simulink model "Controller_Design_Simulink"  (R2025b)
settings: Solver=ode45  StartTime=0.0  StopTime=1  RelTol=1e-10
InitFcn:
  | load("simulink_data.mat")
StartFcn:
  | load("simulink_data.mat")
values from neighbouring files (symbols this model uses):
  A_2 = 1    [Controller_Design.m]    (also in DISTURBANCE TOLERANCE ANALYSYS 2.B.III.mat; Disturbance_tolerance_2.B.I.mat; simulink_data.mat)
  denC = [1 0 0 0]    [simulink_data.mat]
  denFf = [1 4442.21201218 9869604.40109 0]    [simulink_data.mat]
  denFr = 1    [simulink_data.mat]
  denH = [1 88.8576587632 286218.527632 12540956.142 19919185025.5]    [simulink_data.mat]
  denP = [1 1461.98844298 0.0730994152047]    [simulink_data.mat]
  f = 55    [Controller_Design.m]    (also in DISTURBANCE TOLERANCE ANALYSYS 2.B.III.mat = 60; Disturbance_tolerance_2.B.I.mat = 60; simulink_data.mat)
  numC = [0 -1 -4 -4]    [simulink_data.mat]
  numFf = [0 -1731.54607852 -2531500.35528 -126.57500574]    [simulink_data.mat]
  numFr = 1    [simulink_data.mat]
  numH = [1 0 282270.685871 0 19919185025.5]    [simulink_data.mat]
  numP = [0 -5699.87973381 0]    [simulink_data.mat]
libraries: simulink x1
settings Model: Creator=jacop  LastModifiedBy=jacop

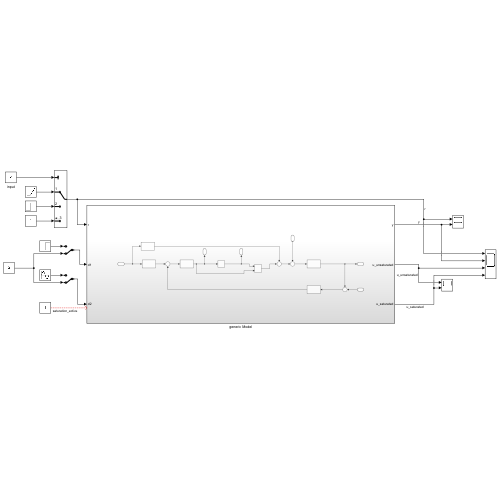
[thumbnail: Simulink's stored preview of the top-level diagram]
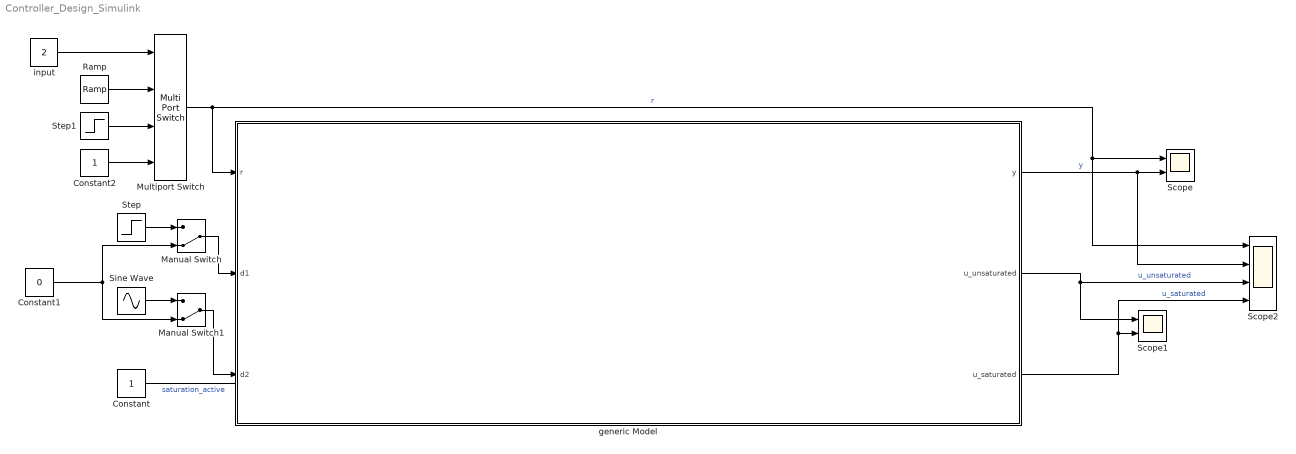
== system Controller_Design_Simulink ==
  Constant : Constant
  Constant1 : Constant  Value=0
  Constant2 : Constant
  Manual Switch : ManualSwitch  CurrentSetting=0
  Manual Switch1 : ManualSwitch  CurrentSetting=0
  Multiport Switch : MultiPortSwitch  SaturateOnIntegerOverflow=off  InputSameDT=off
  Ramp : simulink/Sources/Ramp  slope=1  start=0  InitialOutput=0
  Scope : Scope  NumInputPorts=2
      settings: ActiveDisplayYMinimum=9.9997548415478573E+9  ActiveDisplayYMaximum=1.0000142907162624E+10
  Scope1 : Scope  NumInputPorts=2
      settings: ActiveDisplayYMinimum=-18924.681476074558  ActiveDisplayYMaximum=2102.7423862305059
  Scope2 : Scope  NumInputPorts=4
      settings: ActiveDisplayYMinimum=-50312.130787861315  ActiveDisplayYMaximum=446718.69500859728  DataLoggingVariableName=ScopeData2
  Sine Wave : Sin  Amplitude=A_2  Frequency=2*pi*f  SampleTime=0
  Step : Step  SampleTime=0
  Step1 : Step  Time=0  After=1e7  SampleTime=0
  generic Model : Subsystem
  input : Constant  Value=2
  wires:
  Ramp/1 -> Multiport Switch/2
  Step/1 -> Manual Switch/1
  generic Model/1(y) -> Scope2/2, Scope/2  "y"
  Constant/1 -> ?  "saturation_active"
  generic Model/2(u_unsaturated) -> Scope1/1, Scope2/3  "u_unsaturated"
  generic Model/3(u_saturated) -> Scope2/4, Scope1/2  "u_saturated"
  Constant1/1 -> Manual Switch/2, Manual Switch1/2
  Multiport Switch/1 -> Scope2/1, Scope/1, generic Model/1(r)  "r"
  input/1 -> Multiport Switch/1
  Constant2/1 -> Multiport Switch/4
  Step1/1 -> Multiport Switch/3
  Sine Wave/1 -> Manual Switch1/1
  Manual Switch/1 -> generic Model/2(d1)
  Manual Switch1/1 -> generic Model/3(d2)

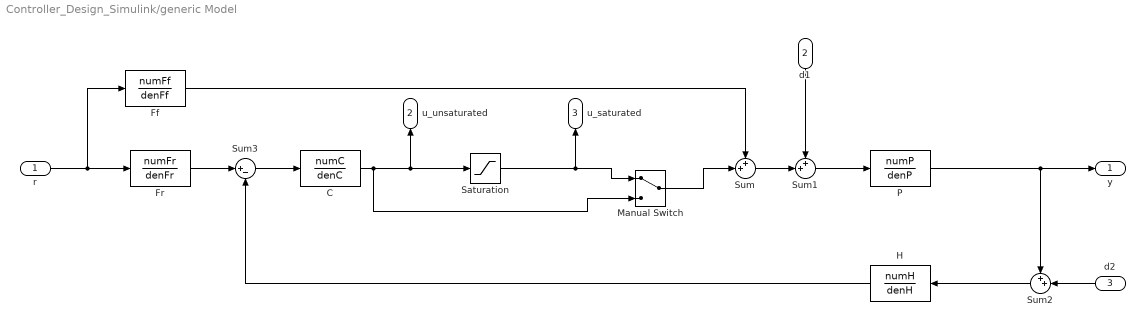
== system Controller_Design_Simulink/generic Model ==
  r : Inport
  d1 : Inport  Port=2
  d2 : Inport  Port=3
  C : TransferFcn  Numerator=numC  Denominator=denC
  Ff : TransferFcn  Numerator=numFf  Denominator=denFf
  Fr : TransferFcn  Numerator=numFr  Denominator=denFr
  H : TransferFcn  Numerator=numH  Denominator=denH
  Manual Switch : ManualSwitch
  P : TransferFcn  Numerator=numP  Denominator=denP
  Saturation : Saturate  UpperLimit=5*1000  LowerLimit=-5*1000
  Sum : Sum  Inputs=++|
  Sum1 : Sum  Inputs=++|
  Sum2 : Sum  Inputs=++|
  Sum3 : Sum  Inputs=|+-
  y : Outport
  u_unsaturated : Outport  Port=2
  u_saturated : Outport  Port=3
  wires:
  Sum2/1 -> H/1
  Ff/1 -> Sum/1
  r/1 -> Fr/1, Ff/1
  Sum1/1 -> P/1
  Sum/1 -> Sum1/2
  Sum3/1 -> C/1
  P/1 -> y/1, Sum2/1
  Fr/1 -> Sum3/1
  d2/1 -> Sum2/2
  H/1 -> Sum3/2
  d1/1 -> Sum1/1
  Manual Switch/1 -> Sum/2
  C/1 -> Saturation/1, u_unsaturated/1, Manual Switch/2
  Saturation/1 -> Manual Switch/1, u_saturated/1
